simulink model "EiH_VFC_Renew_R2021b"  (R2021b)
settings: Solver=ode4  StartTime=0.0  StopTime=30  FixedStep=0.01  RelTol=1e-3
values from neighbouring files (symbols this model uses):
  denomi_threshold = 1e-8    (= 1e-08)    [param_EiH_VFC.m]
  Keo1 = Keo_Gain    (= 0.5)    [param_EiH_VFC.m]
  Keo2 = Keo_Gain    (= 0.5)    [param_EiH_VFC.m]
  Keo3 = Keo_Gain    (= 0.5)    [param_EiH_VFC.m]
  Keo4 = Keo_Gain    (= 0.5)    [param_EiH_VFC.m]
  Keo5 = Keo_Gain    (= 0.5)    [param_EiH_VFC.m]
  Keo6 = Keo_Gain    (= 0.5)    [param_EiH_VFC.m]
  pco_bar_init = pco_init + [0.15; 0.3; -0.1]    [param_EiH_VFC.m]
  pco_init = [0.0; 0.0; -1.0]    [param_EiH_VFC.m]
  Pinho_Para = [0; 0; 0; lambda_mx; lambda_my]    [param_EiH_VFC.m]
  po = [xo1; yo1; zo1; xo2; yo2; zo2; xo3; yo3; zo3; xo4; yo4; zo4]    [param_EiH_VFC.m]
  pzeta_wo_init = [pwo_init;zetawo_init]    [param_EiH_VFC.m]
  R_threshold = 1e-8    (= 1e-08)    [param_EiH_VFC.m]
  Rco_bar_init = Rfromxi(zetaco_bar_init)    [param_EiH_VFC.m]
  Rco_init = Rfromxi(zetaco_init)    [param_EiH_VFC.m]
  sx = -1.02500e5    (= -102500)    [param_EiH_VFC.m]
  sy = -1.02500e5    (= -102500)    [param_EiH_VFC.m]
  zeta_threshold = 1e-8    (= 1e-08)    [param_EiH_VFC.m]
undefined symbols (not defined in the file or in its folder): Angle, Axis, Km1, Km2, Km3, Km4, Km5, Km6, magnitude, pzeta_md
libraries: dspmtrx3 x2, robotcorelib x1, vrlib x1
(part 4 of 4)

== system EiH_VFC_Renew_R2021b/Image Jacobian fco/Image Jacobian/J3/Ji_Left/Ji_Left_x ==
  pci_bar : Inport
  Pinho_Para : Inport  Port=2
  Demux2 : Demux  Outputs=3
      settings: DisplayOption=none
  Demux4 : Demux  Outputs=5
      settings: DisplayOption=none
  Product1 : Product  Inputs=4  InputSameDT=on  SaturateOnIntegerOverflow=on  OutDataTypeStr=Inherit: Same as first input
  Product2 : Product  Inputs=/  InputSameDT=on  SaturateOnIntegerOverflow=on  OutDataTypeStr=Inherit: Same as first input
  Product3 : Product  Inputs=4  InputSameDT=on  SaturateOnIntegerOverflow=on  OutDataTypeStr=Inherit: Same as first input
  Sum : Sum  InputSameDT=on  SaturateOnIntegerOverflow=on  OutDataTypeStr=Inherit: Same as first input
  Terminator{,1..4} (5 alike) : Terminator
  constant1 : Constant  Value=[0;1]  VectorParams1D=off
  constant2 : Constant  Value=[1;0]  VectorParams1D=off
  constant3 : Constant  VectorParams1D=off
  constant4 : Constant  Value=0  VectorParams1D=off
  denomi_threshold : Subsystem
  Ji_Left_x : Outport  VectorParamsAs1DForOutWhenUnconnected=off
  wires:
  Demux2/3 -> denomi_threshold/1(0)
  Demux4/5 -> Product1/1
  Demux4/3 -> Terminator4/1
  Demux2/1 -> Terminator3/1
  constant4/1 -> Product1/4
  constant3/1 -> Product3/4
  Product2/1 -> Product1/3, Product3/3
  constant1/1 -> Product1/2
  Sum/1 -> Ji_Left_x/1
  Demux4/4 -> Product3/1
  Demux4/2 -> Terminator1/1
  Demux4/1 -> Terminator/1
  denomi_threshold/1(not 0) -> Product2/1
  constant2/1 -> Product3/2
  Product3/1 -> Sum/1
  Product1/1 -> Sum/2
  pci_bar/1 -> Demux2/1
  Pinho_Para/1 -> Demux4/1
  Demux2/2 -> Terminator2/1

== system EiH_VFC_Renew_R2021b/Image Jacobian fco/Image Jacobian/J3/Ji_Left/Ji_Left_y ==
  pci_bar : Inport
  Pinho_Para : Inport  Port=2
  Demux2 : Demux  Outputs=3
      settings: DisplayOption=none
  Demux4 : Demux  Outputs=5
      settings: DisplayOption=none
  Product1 : Product  Inputs=4  InputSameDT=on  SaturateOnIntegerOverflow=on  OutDataTypeStr=Inherit: Same as first input
  Product2 : Product  Inputs=/  InputSameDT=on  SaturateOnIntegerOverflow=on  OutDataTypeStr=Inherit: Same as first input
  Product3 : Product  Inputs=4  InputSameDT=on  SaturateOnIntegerOverflow=on  OutDataTypeStr=Inherit: Same as first input
  Sum : Sum  InputSameDT=on  SaturateOnIntegerOverflow=on  OutDataTypeStr=Inherit: Same as first input
  Terminator{,1..4} (5 alike) : Terminator
  constant1 : Constant  Value=[0;1]  VectorParams1D=off
  constant2 : Constant  Value=[1;0]  VectorParams1D=off
  constant3 : Constant  Value=0  VectorParams1D=off
  constant4 : Constant  VectorParams1D=off
  denomi_threshold : Subsystem
  Ji_Left_y : Outport  VectorParamsAs1DForOutWhenUnconnected=off
  wires:
  Product1/1 -> Sum/2
  Product3/1 -> Sum/1
  constant2/1 -> Product3/2
  denomi_threshold/1(not 0) -> Product2/1
  Demux4/1 -> Terminator/1
  Demux4/2 -> Terminator1/1
  Demux4/4 -> Product3/1
  pci_bar/1 -> Demux2/1
  Sum/1 -> Ji_Left_y/1
  Pinho_Para/1 -> Demux4/1
  constant1/1 -> Product1/2
  Product2/1 -> Product3/3, Product1/3
  constant3/1 -> Product3/4
  constant4/1 -> Product1/4
  Demux2/1 -> Terminator3/1
  Demux4/3 -> Terminator4/1
  Demux4/5 -> Product1/1
  Demux2/3 -> denomi_threshold/1(0)
  Demux2/2 -> Terminator2/1

== system EiH_VFC_Renew_R2021b/Image Jacobian fco/Image Jacobian/J3/Ji_Left/Ji_Left_z ==
  pci_bar : Inport
  Pinho_Para : Inport  Port=2
  Demux2 : Demux  Outputs=3
      settings: DisplayOption=none
  Demux4 : Demux  Outputs=5
      settings: DisplayOption=none
  Product1 : Product  Inputs=5  InputSameDT=on  SaturateOnIntegerOverflow=on  OutDataTypeStr=Inherit: Same as first input
  Product2 : Product  Inputs=/  InputSameDT=on  SaturateOnIntegerOverflow=on  OutDataTypeStr=Inherit: Same as first input
  Product3 : Product  Inputs=5  InputSameDT=on  SaturateOnIntegerOverflow=on  OutDataTypeStr=Inherit: Same as first input
  Sum : Sum  Inputs=--  InputSameDT=on  SaturateOnIntegerOverflow=on  OutDataTypeStr=Inherit: Same as first input
  Terminator : Terminator
  Terminator1 : Terminator
  Terminator2 : Terminator
  constant1 : Constant  Value=[0;1]  VectorParams1D=off
  constant2 : Constant  Value=[1;0]  VectorParams1D=off
  denomi_threshold : Subsystem
  Ji_Left_z : Outport  VectorParamsAs1DForOutWhenUnconnected=off
  wires:
  Demux2/1 -> Product3/2
  Product2/1 -> Product3/5, Product3/4, Product1/4, Product1/5
  constant1/1 -> Product1/3
  Pinho_Para/1 -> Demux4/1
  Sum/1 -> Ji_Left_z/1
  pci_bar/1 -> Demux2/1
  Demux4/4 -> Product3/1
  Demux4/2 -> Terminator1/1
  Demux4/1 -> Terminator/1
  denomi_threshold/1(not 0) -> Product2/1
  constant2/1 -> Product3/3
  Product3/1 -> Sum/1
  Product1/1 -> Sum/2
  Demux4/3 -> Terminator2/1
  Demux4/5 -> Product1/1
  Demux2/3 -> denomi_threshold/1(0)
  Demux2/2 -> Product1/2

== system EiH_VFC_Renew_R2021b/Image Jacobian fco/Image Jacobian/J3/Ji_Right/wedge ==
  "[3x1]" : Inport
  Product1 : Product  InputSameDT=on  SaturateOnIntegerOverflow=on  OutDataTypeStr=Inherit: Same as first input
  Product2 : Product  InputSameDT=on  SaturateOnIntegerOverflow=on  OutDataTypeStr=Inherit: Same as first input
  Product3 : Product  InputSameDT=on  SaturateOnIntegerOverflow=on  OutDataTypeStr=Inherit: Same as first input
  Sum : Sum  Inputs=+++  InputSameDT=on  SaturateOnIntegerOverflow=on  OutDataTypeStr=Inherit: Same as first input
  Xaxis : Constant  Value=[0 0 0;0 0 -1;0 1 0]  VectorParams1D=off
  Yaxis : Constant  Value=[0 0 1;0 0 0;-1 0 0]  VectorParams1D=off
  Zaxis : Constant  Value=[0 -1 0;1 0 0;0 0 0]  VectorParams1D=off
  x : Gain  Gain=[1 0 0]  Multiplication=Matrix(K*u)  SaturateOnIntegerOverflow=on  OutDataTypeStr=Inherit: Same as input  ParamDataTypeStr=Inherit: Same as input
  y : Gain  Gain=[0 1 0]  Multiplication=Matrix(K*u)  SaturateOnIntegerOverflow=on  OutDataTypeStr=Inherit: Same as input  ParamDataTypeStr=Inherit: Same as input
  z : Gain  Gain=[0 0 1]  Multiplication=Matrix(K*u)  SaturateOnIntegerOverflow=on  OutDataTypeStr=Inherit: Same as input  ParamDataTypeStr=Inherit: Same as input
  "[3x3]" : Outport  VectorParamsAs1DForOutWhenUnconnected=off
  wires:
  Zaxis/1 -> Product1/2
  z/1 -> Product1/1
  Xaxis/1 -> Product2/2
  x/1 -> Product2/1
  Yaxis/1 -> Product3/2
  y/1 -> Product3/1
  "[3x1]"/1 -> y/1, x/1, z/1
  Product3/1 -> Sum/2
  Product2/1 -> Sum/1
  Product1/1 -> Sum/3
  Sum/1 -> "[3x3]"/1

== system EiH_VFC_Renew_R2021b/Image Jacobian fco/Image Jacobian/J4/Ji_Left/Ji_Left_x ==
  pci_bar : Inport
  Pinho_Para : Inport  Port=2
  Demux2 : Demux  Outputs=3
      settings: DisplayOption=none
  Demux4 : Demux  Outputs=5
      settings: DisplayOption=none
  Product1 : Product  Inputs=4  InputSameDT=on  SaturateOnIntegerOverflow=on  OutDataTypeStr=Inherit: Same as first input
  Product2 : Product  Inputs=/  InputSameDT=on  SaturateOnIntegerOverflow=on  OutDataTypeStr=Inherit: Same as first input
  Product3 : Product  Inputs=4  InputSameDT=on  SaturateOnIntegerOverflow=on  OutDataTypeStr=Inherit: Same as first input
  Sum : Sum  InputSameDT=on  SaturateOnIntegerOverflow=on  OutDataTypeStr=Inherit: Same as first input
  Terminator{,1..4} (5 alike) : Terminator
  constant1 : Constant  Value=[0;1]  VectorParams1D=off
  constant2 : Constant  Value=[1;0]  VectorParams1D=off
  constant3 : Constant  VectorParams1D=off
  constant4 : Constant  Value=0  VectorParams1D=off
  denomi_threshold : Subsystem
  Ji_Left_x : Outport  VectorParamsAs1DForOutWhenUnconnected=off
  wires:
  Demux2/3 -> denomi_threshold/1(0)
  Demux4/5 -> Product1/1
  Demux4/3 -> Terminator4/1
  Demux2/1 -> Terminator3/1
  constant4/1 -> Product1/4
  constant3/1 -> Product3/4
  Product2/1 -> Product1/3, Product3/3
  constant1/1 -> Product1/2
  Sum/1 -> Ji_Left_x/1
  Demux4/4 -> Product3/1
  Demux4/2 -> Terminator1/1
  Demux4/1 -> Terminator/1
  denomi_threshold/1(not 0) -> Product2/1
  constant2/1 -> Product3/2
  Product3/1 -> Sum/1
  Product1/1 -> Sum/2
  pci_bar/1 -> Demux2/1
  Pinho_Para/1 -> Demux4/1
  Demux2/2 -> Terminator2/1

== system EiH_VFC_Renew_R2021b/Image Jacobian fco/Image Jacobian/J4/Ji_Left/Ji_Left_y ==
  pci_bar : Inport
  Pinho_Para : Inport  Port=2
  Demux2 : Demux  Outputs=3
      settings: DisplayOption=none
  Demux4 : Demux  Outputs=5
      settings: DisplayOption=none
  Product1 : Product  Inputs=4  InputSameDT=on  SaturateOnIntegerOverflow=on  OutDataTypeStr=Inherit: Same as first input
  Product2 : Product  Inputs=/  InputSameDT=on  SaturateOnIntegerOverflow=on  OutDataTypeStr=Inherit: Same as first input
  Product3 : Product  Inputs=4  InputSameDT=on  SaturateOnIntegerOverflow=on  OutDataTypeStr=Inherit: Same as first input
  Sum : Sum  InputSameDT=on  SaturateOnIntegerOverflow=on  OutDataTypeStr=Inherit: Same as first input
  Terminator{,1..4} (5 alike) : Terminator
  constant1 : Constant  Value=[0;1]  VectorParams1D=off
  constant2 : Constant  Value=[1;0]  VectorParams1D=off
  constant3 : Constant  Value=0  VectorParams1D=off
  constant4 : Constant  VectorParams1D=off
  denomi_threshold : Subsystem
  Ji_Left_y : Outport  VectorParamsAs1DForOutWhenUnconnected=off
  wires:
  Product1/1 -> Sum/2
  Product3/1 -> Sum/1
  constant2/1 -> Product3/2
  denomi_threshold/1(not 0) -> Product2/1
  Demux4/1 -> Terminator/1
  Demux4/2 -> Terminator1/1
  Demux4/4 -> Product3/1
  pci_bar/1 -> Demux2/1
  Sum/1 -> Ji_Left_y/1
  Pinho_Para/1 -> Demux4/1
  constant1/1 -> Product1/2
  Product2/1 -> Product3/3, Product1/3
  constant3/1 -> Product3/4
  constant4/1 -> Product1/4
  Demux2/1 -> Terminator3/1
  Demux4/3 -> Terminator4/1
  Demux4/5 -> Product1/1
  Demux2/3 -> denomi_threshold/1(0)
  Demux2/2 -> Terminator2/1

== system EiH_VFC_Renew_R2021b/Image Jacobian fco/Image Jacobian/J4/Ji_Left/Ji_Left_z ==
  pci_bar : Inport
  Pinho_Para : Inport  Port=2
  Demux2 : Demux  Outputs=3
      settings: DisplayOption=none
  Demux4 : Demux  Outputs=5
      settings: DisplayOption=none
  Product1 : Product  Inputs=5  InputSameDT=on  SaturateOnIntegerOverflow=on  OutDataTypeStr=Inherit: Same as first input
  Product2 : Product  Inputs=/  InputSameDT=on  SaturateOnIntegerOverflow=on  OutDataTypeStr=Inherit: Same as first input
  Product3 : Product  Inputs=5  InputSameDT=on  SaturateOnIntegerOverflow=on  OutDataTypeStr=Inherit: Same as first input
  Sum : Sum  Inputs=--  InputSameDT=on  SaturateOnIntegerOverflow=on  OutDataTypeStr=Inherit: Same as first input
  Terminator : Terminator
  Terminator1 : Terminator
  Terminator2 : Terminator
  constant1 : Constant  Value=[0;1]  VectorParams1D=off
  constant2 : Constant  Value=[1;0]  VectorParams1D=off
  denomi_threshold : Subsystem
  Ji_Left_z : Outport  VectorParamsAs1DForOutWhenUnconnected=off
  wires:
  Demux2/1 -> Product3/2
  Product2/1 -> Product3/5, Product3/4, Product1/4, Product1/5
  constant1/1 -> Product1/3
  Pinho_Para/1 -> Demux4/1
  Sum/1 -> Ji_Left_z/1
  pci_bar/1 -> Demux2/1
  Demux4/4 -> Product3/1
  Demux4/2 -> Terminator1/1
  Demux4/1 -> Terminator/1
  denomi_threshold/1(not 0) -> Product2/1
  constant2/1 -> Product3/3
  Product3/1 -> Sum/1
  Product1/1 -> Sum/2
  Demux4/3 -> Terminator2/1
  Demux4/5 -> Product1/1
  Demux2/3 -> denomi_threshold/1(0)
  Demux2/2 -> Product1/2

== system EiH_VFC_Renew_R2021b/Image Jacobian fco/Image Jacobian/J4/Ji_Right/wedge ==
  "[3x1]" : Inport
  Product1 : Product  InputSameDT=on  SaturateOnIntegerOverflow=on  OutDataTypeStr=Inherit: Same as first input
  Product2 : Product  InputSameDT=on  SaturateOnIntegerOverflow=on  OutDataTypeStr=Inherit: Same as first input
  Product3 : Product  InputSameDT=on  SaturateOnIntegerOverflow=on  OutDataTypeStr=Inherit: Same as first input
  Sum : Sum  Inputs=+++  InputSameDT=on  SaturateOnIntegerOverflow=on  OutDataTypeStr=Inherit: Same as first input
  Xaxis : Constant  Value=[0 0 0;0 0 -1;0 1 0]  VectorParams1D=off
  Yaxis : Constant  Value=[0 0 1;0 0 0;-1 0 0]  VectorParams1D=off
  Zaxis : Constant  Value=[0 -1 0;1 0 0;0 0 0]  VectorParams1D=off
  x : Gain  Gain=[1 0 0]  Multiplication=Matrix(K*u)  SaturateOnIntegerOverflow=on  OutDataTypeStr=Inherit: Same as input  ParamDataTypeStr=Inherit: Same as input
  y : Gain  Gain=[0 1 0]  Multiplication=Matrix(K*u)  SaturateOnIntegerOverflow=on  OutDataTypeStr=Inherit: Same as input  ParamDataTypeStr=Inherit: Same as input
  z : Gain  Gain=[0 0 1]  Multiplication=Matrix(K*u)  SaturateOnIntegerOverflow=on  OutDataTypeStr=Inherit: Same as input  ParamDataTypeStr=Inherit: Same as input
  "[3x3]" : Outport  VectorParamsAs1DForOutWhenUnconnected=off
  wires:
  Zaxis/1 -> Product1/2
  z/1 -> Product1/1
  Xaxis/1 -> Product2/2
  x/1 -> Product2/1
  Yaxis/1 -> Product3/2
  y/1 -> Product3/1
  "[3x1]"/1 -> y/1, x/1, z/1
  Product3/1 -> Sum/2
  Product2/1 -> Sum/1
  Product1/1 -> Sum/3
  Sum/1 -> "[3x3]"/1

== system EiH_VFC_Renew_R2021b/Vision Camera fco/ fcq /fcq1/make fcqi/denomi_threshold ==
  0 : Inport
  Abs : Abs  SaturateOnIntegerOverflow=on
  Switch : Switch  Threshold=denomi_threshold  SaturateOnIntegerOverflow=on  InputSameDT=on
  denomi_threshold : Constant  Value=denomi_threshold  VectorParams1D=off
  not 0 : Outport  VectorParamsAs1DForOutWhenUnconnected=off
  wires:
  Switch/1 -> not 0/1
  denomi_threshold/1 -> Switch/3
  0/1 -> Switch/1, Abs/1
  Abs/1 -> Switch/2

== system EiH_VFC_Renew_R2021b/Vision Camera fco/ fcq /fcq2/make fcqi/denomi_threshold ==
  0 : Inport
  Abs : Abs  SaturateOnIntegerOverflow=on
  Switch : Switch  Threshold=denomi_threshold  SaturateOnIntegerOverflow=on  InputSameDT=on
  denomi_threshold : Constant  Value=denomi_threshold  VectorParams1D=off
  not 0 : Outport  VectorParamsAs1DForOutWhenUnconnected=off
  wires:
  Switch/1 -> not 0/1
  denomi_threshold/1 -> Switch/3
  0/1 -> Switch/1, Abs/1
  Abs/1 -> Switch/2

== system EiH_VFC_Renew_R2021b/Vision Camera fco/ fcq /fcq3/make fcqi/denomi_threshold ==
  0 : Inport
  Abs : Abs  SaturateOnIntegerOverflow=on
  Switch : Switch  Threshold=denomi_threshold  SaturateOnIntegerOverflow=on  InputSameDT=on
  denomi_threshold : Constant  Value=denomi_threshold  VectorParams1D=off
  not 0 : Outport  VectorParamsAs1DForOutWhenUnconnected=off
  wires:
  Switch/1 -> not 0/1
  denomi_threshold/1 -> Switch/3
  0/1 -> Switch/1, Abs/1
  Abs/1 -> Switch/2

== system EiH_VFC_Renew_R2021b/Vision Camera fco/ fcq /fcq4/make fcqi/denomi_threshold ==
  0 : Inport
  Abs : Abs  SaturateOnIntegerOverflow=on
  Switch : Switch  Threshold=denomi_threshold  SaturateOnIntegerOverflow=on  InputSameDT=on
  denomi_threshold : Constant  Value=denomi_threshold  VectorParams1D=off
  not 0 : Outport  VectorParamsAs1DForOutWhenUnconnected=off
  wires:
  Switch/1 -> not 0/1
  denomi_threshold/1 -> Switch/3
  0/1 -> Switch/1, Abs/1
  Abs/1 -> Switch/2

== system EiH_VFC_Renew_R2021b/Vision Camera fco/make pzeta co/Rco -> zeta_co/e_R(R)/sk(R) ==
  R : Inport
  Gain : Gain  Gain=1/2  SaturateOnIntegerOverflow=on  OutDataTypeStr=Inherit: Same as input  ParamDataTypeStr=Inherit: Same as input
  Math Function2 : Math  Operator=transpose  SignedPower=on  SaturateOnIntegerOverflow=on
  Sum : Sum  Inputs=|+-  InputSameDT=on  SaturateOnIntegerOverflow=on  OutDataTypeStr=Inherit: Same as first input
  sk(R) : Outport  VectorParamsAs1DForOutWhenUnconnected=off
  wires:
  R/1 -> Math Function2/1, Sum/1
  Math Function2/1 -> Sum/2
  Sum/1 -> Gain/1
  Gain/1 -> sk(R)/1

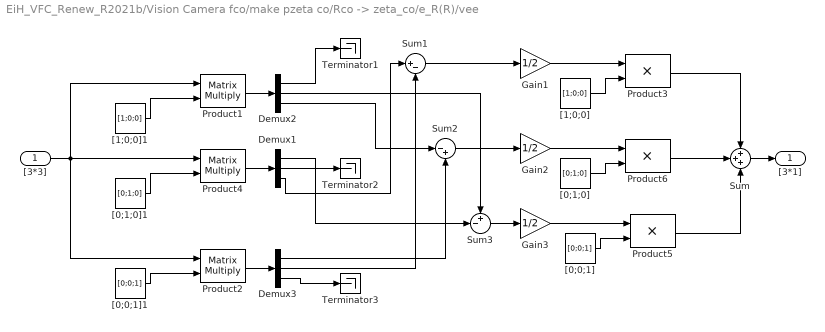
== system EiH_VFC_Renew_R2021b/Vision Camera fco/make pzeta co/Rco -> zeta_co/e_R(R)/vee ==
  "[3*3]" : Inport
  Demux1 : Demux  Outputs=3
      settings: DisplayOption=none
  Demux2 : Demux  Outputs=3
      settings: DisplayOption=none
  Demux3 : Demux  Outputs=3
      settings: DisplayOption=none
  Gain1 : Gain  Gain=1/2  SaturateOnIntegerOverflow=on  OutDataTypeStr=Inherit: Same as input  ParamDataTypeStr=Inherit: Same as input
  Gain2 : Gain  Gain=1/2  SaturateOnIntegerOverflow=on  OutDataTypeStr=Inherit: Same as input  ParamDataTypeStr=Inherit: Same as input
  Gain3 : Gain  Gain=1/2  SaturateOnIntegerOverflow=on  OutDataTypeStr=Inherit: Same as input  ParamDataTypeStr=Inherit: Same as input
  Product1 : Product  Multiplication=Matrix(*)  InputSameDT=on  SaturateOnIntegerOverflow=on  OutDataTypeStr=Inherit: Same as first input
  Product2 : Product  Multiplication=Matrix(*)  InputSameDT=on  SaturateOnIntegerOverflow=on  OutDataTypeStr=Inherit: Same as first input
  Product3 : Product  InputSameDT=on  SaturateOnIntegerOverflow=on  OutDataTypeStr=Inherit: Same as first input
  Product4 : Product  Multiplication=Matrix(*)  InputSameDT=on  SaturateOnIntegerOverflow=on  OutDataTypeStr=Inherit: Same as first input
  Product5 : Product  InputSameDT=on  SaturateOnIntegerOverflow=on  OutDataTypeStr=Inherit: Same as first input
  Product6 : Product  InputSameDT=on  SaturateOnIntegerOverflow=on  OutDataTypeStr=Inherit: Same as first input
  Sum : Sum  Inputs=+++  InputSameDT=on  SaturateOnIntegerOverflow=on  OutDataTypeStr=Inherit: Same as first input
  Sum1 : Sum  Inputs=|+-  InputSameDT=on  SaturateOnIntegerOverflow=on  OutDataTypeStr=Inherit: Same as first input
  Sum2 : Sum  Inputs=|-+  InputSameDT=on  SaturateOnIntegerOverflow=on  OutDataTypeStr=Inherit: Same as first input
  Sum3 : Sum  Inputs=+-|  InputSameDT=on  SaturateOnIntegerOverflow=on  OutDataTypeStr=Inherit: Same as first input
  Terminator1 : Terminator
  Terminator2 : Terminator
  Terminator3 : Terminator
  "[0;0;1]" : Constant  Value=[0;0;1]  VectorParams1D=off
  "[0;0;1]1" : Constant  Value=[0;0;1]  VectorParams1D=off
  "[0;1;0]" : Constant  Value=[0;1;0]  VectorParams1D=off
  "[0;1;0]1" : Constant  Value=[0;1;0]  VectorParams1D=off
  "[1;0;0]" : Constant  Value=[1;0;0]  VectorParams1D=off
  "[1;0;0]1" : Constant  Value=[1;0;0]  VectorParams1D=off
  "[3*1]" : Outport  VectorParamsAs1DForOutWhenUnconnected=off
  wires:
  "[3*3]"/1 -> Product2/1, Product1/1, Product4/1
  "[0;1;0]1"/1 -> Product4/2
  Product4/1 -> Demux1/1
  Demux1/2 -> Terminator2/1
  Demux1/3 -> Sum1/1
  "[1;0;0]1"/1 -> Product1/2
  Product1/1 -> Demux2/1
  Demux2/1 -> Terminator1/1
  "[0;0;1]1"/1 -> Product2/2
  Product2/1 -> Demux3/1
  Demux3/3 -> Terminator3/1
  Demux3/1 -> Sum2/2
  "[1;0;0]"/1 -> Product3/2
  "[0;1;0]"/1 -> Product6/2
  "[0;0;1]"/1 -> Product5/2
  Product6/1 -> Sum/2
  Product5/1 -> Sum/3
  Product3/1 -> Sum/1
  Sum/1 -> "[3*1]"/1
  Sum1/1 -> Gain1/1
  Gain1/1 -> Product3/1
  Demux3/2 -> Sum1/2
  Gain2/1 -> Product6/1
  Gain3/1 -> Product5/1
  Demux2/3 -> Sum2/1
  Sum2/1 -> Gain2/1
  Sum3/1 -> Gain3/1
  Demux2/2 -> Sum3/1
  Demux1/1 -> Sum3/2

== system EiH_VFC_Renew_R2021b/Vision Camera fco/make pzeta co/Rco -> zeta_co/make zeta/3x1 -> 2norm ==
  3x1 : Inport
  Demux : Demux  Outputs=3
      settings: DisplayOption=none
  Math Function : Math  Operator=magnitude^2  SignedPower=on  SaturateOnIntegerOverflow=on
  Math Function1 : Math  Operator=sqrt  SignedPower=on  SaturateOnIntegerOverflow=on
  Sum : Sum  Inputs=+++  InputSameDT=on  SaturateOnIntegerOverflow=on  OutDataTypeStr=Inherit: Same as first input
  2 norm : Outport  VectorParamsAs1DForOutWhenUnconnected=off
  wires:
  Math Function/1 -> Demux/1
  Demux/3 -> Sum/3
  Demux/2 -> Sum/2
  Demux/1 -> Sum/1
  Sum/1 -> Math Function1/1
  Math Function1/1 -> 2 norm/1
  3x1/1 -> Math Function/1

== system EiH_VFC_Renew_R2021b/Vision Camera fco/make pzeta co/Rco -> zeta_co/make zeta/zero check zeta_threshold ==
  In1 : Inport
  Switch : Switch  Threshold=zeta_threshold  SaturateOnIntegerOverflow=on  InputSameDT=on
  norm_eR : Constant  Value=zeta_threshold  VectorParams1D=off
  Out1 : Outport  VectorParamsAs1DForOutWhenUnconnected=off
  wires:
  norm_eR/1 -> Switch/3
  In1/1 -> Switch/1, Switch/2
  Switch/1 -> Out1/1

== system EiH_VFC_Renew_R2021b/make Rco pco/make p_zeta co/make zeta_co/e_R(R)/sk(R) ==
  R : Inport
  Gain : Gain  Gain=1/2  SaturateOnIntegerOverflow=on  OutDataTypeStr=Inherit: Same as input  ParamDataTypeStr=Inherit: Same as input
  Math Function2 : Math  Operator=transpose  SignedPower=on  SaturateOnIntegerOverflow=on
  Sum : Sum  Inputs=|+-  InputSameDT=on  SaturateOnIntegerOverflow=on  OutDataTypeStr=Inherit: Same as first input
  sk(R) : Outport  VectorParamsAs1DForOutWhenUnconnected=off
  wires:
  R/1 -> Math Function2/1, Sum/1
  Math Function2/1 -> Sum/2
  Sum/1 -> Gain/1
  Gain/1 -> sk(R)/1

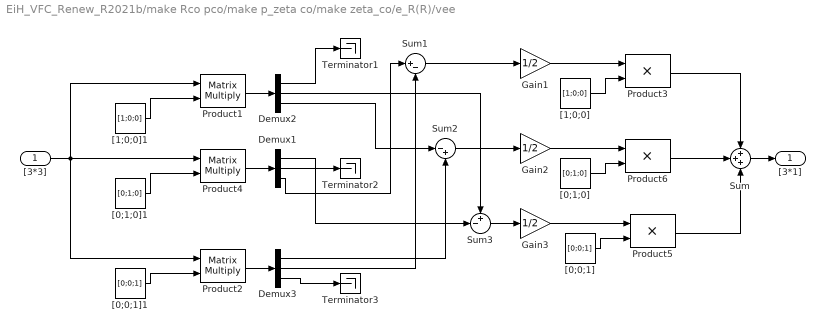
== system EiH_VFC_Renew_R2021b/make Rco pco/make p_zeta co/make zeta_co/e_R(R)/vee ==
  "[3*3]" : Inport
  Demux1 : Demux  Outputs=3
      settings: DisplayOption=none
  Demux2 : Demux  Outputs=3
      settings: DisplayOption=none
  Demux3 : Demux  Outputs=3
      settings: DisplayOption=none
  Gain1 : Gain  Gain=1/2  SaturateOnIntegerOverflow=on  OutDataTypeStr=Inherit: Same as input  ParamDataTypeStr=Inherit: Same as input
  Gain2 : Gain  Gain=1/2  SaturateOnIntegerOverflow=on  OutDataTypeStr=Inherit: Same as input  ParamDataTypeStr=Inherit: Same as input
  Gain3 : Gain  Gain=1/2  SaturateOnIntegerOverflow=on  OutDataTypeStr=Inherit: Same as input  ParamDataTypeStr=Inherit: Same as input
  Product1 : Product  Multiplication=Matrix(*)  InputSameDT=on  SaturateOnIntegerOverflow=on  OutDataTypeStr=Inherit: Same as first input
  Product2 : Product  Multiplication=Matrix(*)  InputSameDT=on  SaturateOnIntegerOverflow=on  OutDataTypeStr=Inherit: Same as first input
  Product3 : Product  InputSameDT=on  SaturateOnIntegerOverflow=on  OutDataTypeStr=Inherit: Same as first input
  Product4 : Product  Multiplication=Matrix(*)  InputSameDT=on  SaturateOnIntegerOverflow=on  OutDataTypeStr=Inherit: Same as first input
  Product5 : Product  InputSameDT=on  SaturateOnIntegerOverflow=on  OutDataTypeStr=Inherit: Same as first input
  Product6 : Product  InputSameDT=on  SaturateOnIntegerOverflow=on  OutDataTypeStr=Inherit: Same as first input
  Sum : Sum  Inputs=+++  InputSameDT=on  SaturateOnIntegerOverflow=on  OutDataTypeStr=Inherit: Same as first input
  Sum1 : Sum  Inputs=|+-  InputSameDT=on  SaturateOnIntegerOverflow=on  OutDataTypeStr=Inherit: Same as first input
  Sum2 : Sum  Inputs=|-+  InputSameDT=on  SaturateOnIntegerOverflow=on  OutDataTypeStr=Inherit: Same as first input
  Sum3 : Sum  Inputs=+-|  InputSameDT=on  SaturateOnIntegerOverflow=on  OutDataTypeStr=Inherit: Same as first input
  Terminator1 : Terminator
  Terminator2 : Terminator
  Terminator3 : Terminator
  "[0;0;1]" : Constant  Value=[0;0;1]  VectorParams1D=off
  "[0;0;1]1" : Constant  Value=[0;0;1]  VectorParams1D=off
  "[0;1;0]" : Constant  Value=[0;1;0]  VectorParams1D=off
  "[0;1;0]1" : Constant  Value=[0;1;0]  VectorParams1D=off
  "[1;0;0]" : Constant  Value=[1;0;0]  VectorParams1D=off
  "[1;0;0]1" : Constant  Value=[1;0;0]  VectorParams1D=off
  "[3*1]" : Outport  VectorParamsAs1DForOutWhenUnconnected=off
  wires:
  "[3*3]"/1 -> Product2/1, Product1/1, Product4/1
  "[0;1;0]1"/1 -> Product4/2
  Product4/1 -> Demux1/1
  Demux1/2 -> Terminator2/1
  Demux1/3 -> Sum1/1
  "[1;0;0]1"/1 -> Product1/2
  Product1/1 -> Demux2/1
  Demux2/1 -> Terminator1/1
  "[0;0;1]1"/1 -> Product2/2
  Product2/1 -> Demux3/1
  Demux3/3 -> Terminator3/1
  Demux3/1 -> Sum2/2
  "[1;0;0]"/1 -> Product3/2
  "[0;1;0]"/1 -> Product6/2
  "[0;0;1]"/1 -> Product5/2
  Product6/1 -> Sum/2
  Product5/1 -> Sum/3
  Product3/1 -> Sum/1
  Sum/1 -> "[3*1]"/1
  Sum1/1 -> Gain1/1
  Gain1/1 -> Product3/1
  Demux3/2 -> Sum1/2
  Gain2/1 -> Product6/1
  Gain3/1 -> Product5/1
  Demux2/3 -> Sum2/1
  Sum2/1 -> Gain2/1
  Sum3/1 -> Gain3/1
  Demux2/2 -> Sum3/1
  Demux1/1 -> Sum3/2

== system EiH_VFC_Renew_R2021b/make Rco pco/make p_zeta co/make zeta_co/make zeta/3x1 -> 2norm ==
  3x1 : Inport
  Demux : Demux  Outputs=3
      settings: DisplayOption=none
  Math Function : Math  Operator=magnitude^2  SignedPower=on  SaturateOnIntegerOverflow=on
  Math Function1 : Math  Operator=sqrt  SignedPower=on  SaturateOnIntegerOverflow=on
  Sum : Sum  Inputs=+++  InputSameDT=on  SaturateOnIntegerOverflow=on  OutDataTypeStr=Inherit: Same as first input
  2 norm : Outport  VectorParamsAs1DForOutWhenUnconnected=off
  wires:
  Math Function/1 -> Demux/1
  Demux/3 -> Sum/3
  Demux/2 -> Sum/2
  Demux/1 -> Sum/1
  Sum/1 -> Math Function1/1
  Math Function1/1 -> 2 norm/1
  3x1/1 -> Math Function/1

== system EiH_VFC_Renew_R2021b/make Rco pco/make p_zeta co/make zeta_co/make zeta/zero check zeta_threshold ==
  In1 : Inport
  Switch : Switch  Threshold=zeta_threshold  SaturateOnIntegerOverflow=on  InputSameDT=on
  norm_eR : Constant  Value=zeta_threshold  VectorParams1D=off
  Out1 : Outport  VectorParamsAs1DForOutWhenUnconnected=off
  wires:
  norm_eR/1 -> Switch/3
  In1/1 -> Switch/1, Switch/2
  Switch/1 -> Out1/1

== system EiH_VFC_Renew_R2021b/Image Jacobian fco/Image Jacobian/J1/Ji_Left/Ji_Left_x/denomi_threshold ==
  0 : Inport
  Abs : Abs  SaturateOnIntegerOverflow=on
  Switch : Switch  Threshold=denomi_threshold  SaturateOnIntegerOverflow=on  InputSameDT=on
  denomi_threshold : Constant  Value=denomi_threshold  VectorParams1D=off
  not 0 : Outport  VectorParamsAs1DForOutWhenUnconnected=off
  wires:
  Switch/1 -> not 0/1
  denomi_threshold/1 -> Switch/3
  0/1 -> Switch/1, Abs/1
  Abs/1 -> Switch/2

== system EiH_VFC_Renew_R2021b/Image Jacobian fco/Image Jacobian/J1/Ji_Left/Ji_Left_y/denomi_threshold ==
  0 : Inport
  Abs : Abs  SaturateOnIntegerOverflow=on
  Switch : Switch  Threshold=denomi_threshold  SaturateOnIntegerOverflow=on  InputSameDT=on
  denomi_threshold : Constant  Value=denomi_threshold  VectorParams1D=off
  not 0 : Outport  VectorParamsAs1DForOutWhenUnconnected=off
  wires:
  Abs/1 -> Switch/2
  0/1 -> Abs/1, Switch/1
  denomi_threshold/1 -> Switch/3
  Switch/1 -> not 0/1

== system EiH_VFC_Renew_R2021b/Image Jacobian fco/Image Jacobian/J1/Ji_Left/Ji_Left_z/denomi_threshold ==
  0 : Inport
  Abs : Abs  SaturateOnIntegerOverflow=on
  Switch : Switch  Threshold=denomi_threshold  SaturateOnIntegerOverflow=on  InputSameDT=on
  denomi_threshold : Constant  Value=denomi_threshold  VectorParams1D=off
  not 0 : Outport  VectorParamsAs1DForOutWhenUnconnected=off
  wires:
  Switch/1 -> not 0/1
  denomi_threshold/1 -> Switch/3
  0/1 -> Switch/1, Abs/1
  Abs/1 -> Switch/2

== system EiH_VFC_Renew_R2021b/Image Jacobian fco/Image Jacobian/J2/Ji_Left/Ji_Left_x/denomi_threshold ==
  0 : Inport
  Abs : Abs  SaturateOnIntegerOverflow=on
  Switch : Switch  Threshold=denomi_threshold  SaturateOnIntegerOverflow=on  InputSameDT=on
  denomi_threshold : Constant  Value=denomi_threshold  VectorParams1D=off
  not 0 : Outport  VectorParamsAs1DForOutWhenUnconnected=off
  wires:
  Switch/1 -> not 0/1
  denomi_threshold/1 -> Switch/3
  0/1 -> Switch/1, Abs/1
  Abs/1 -> Switch/2

== system EiH_VFC_Renew_R2021b/Image Jacobian fco/Image Jacobian/J2/Ji_Left/Ji_Left_y/denomi_threshold ==
  0 : Inport
  Abs : Abs  SaturateOnIntegerOverflow=on
  Switch : Switch  Threshold=denomi_threshold  SaturateOnIntegerOverflow=on  InputSameDT=on
  denomi_threshold : Constant  Value=denomi_threshold  VectorParams1D=off
  not 0 : Outport  VectorParamsAs1DForOutWhenUnconnected=off
  wires:
  Abs/1 -> Switch/2
  0/1 -> Abs/1, Switch/1
  denomi_threshold/1 -> Switch/3
  Switch/1 -> not 0/1

== system EiH_VFC_Renew_R2021b/Image Jacobian fco/Image Jacobian/J2/Ji_Left/Ji_Left_z/denomi_threshold ==
  0 : Inport
  Abs : Abs  SaturateOnIntegerOverflow=on
  Switch : Switch  Threshold=denomi_threshold  SaturateOnIntegerOverflow=on  InputSameDT=on
  denomi_threshold : Constant  Value=denomi_threshold  VectorParams1D=off
  not 0 : Outport  VectorParamsAs1DForOutWhenUnconnected=off
  wires:
  Switch/1 -> not 0/1
  denomi_threshold/1 -> Switch/3
  0/1 -> Switch/1, Abs/1
  Abs/1 -> Switch/2

== system EiH_VFC_Renew_R2021b/Image Jacobian fco/Image Jacobian/J3/Ji_Left/Ji_Left_x/denomi_threshold ==
  0 : Inport
  Abs : Abs  SaturateOnIntegerOverflow=on
  Switch : Switch  Threshold=denomi_threshold  SaturateOnIntegerOverflow=on  InputSameDT=on
  denomi_threshold : Constant  Value=denomi_threshold  VectorParams1D=off
  not 0 : Outport  VectorParamsAs1DForOutWhenUnconnected=off
  wires:
  Switch/1 -> not 0/1
  denomi_threshold/1 -> Switch/3
  0/1 -> Switch/1, Abs/1
  Abs/1 -> Switch/2

== system EiH_VFC_Renew_R2021b/Image Jacobian fco/Image Jacobian/J3/Ji_Left/Ji_Left_y/denomi_threshold ==
  0 : Inport
  Abs : Abs  SaturateOnIntegerOverflow=on
  Switch : Switch  Threshold=denomi_threshold  SaturateOnIntegerOverflow=on  InputSameDT=on
  denomi_threshold : Constant  Value=denomi_threshold  VectorParams1D=off
  not 0 : Outport  VectorParamsAs1DForOutWhenUnconnected=off
  wires:
  Abs/1 -> Switch/2
  0/1 -> Abs/1, Switch/1
  denomi_threshold/1 -> Switch/3
  Switch/1 -> not 0/1

== system EiH_VFC_Renew_R2021b/Image Jacobian fco/Image Jacobian/J3/Ji_Left/Ji_Left_z/denomi_threshold ==
  0 : Inport
  Abs : Abs  SaturateOnIntegerOverflow=on
  Switch : Switch  Threshold=denomi_threshold  SaturateOnIntegerOverflow=on  InputSameDT=on
  denomi_threshold : Constant  Value=denomi_threshold  VectorParams1D=off
  not 0 : Outport  VectorParamsAs1DForOutWhenUnconnected=off
  wires:
  Switch/1 -> not 0/1
  denomi_threshold/1 -> Switch/3
  0/1 -> Switch/1, Abs/1
  Abs/1 -> Switch/2

== system EiH_VFC_Renew_R2021b/Image Jacobian fco/Image Jacobian/J4/Ji_Left/Ji_Left_x/denomi_threshold ==
  0 : Inport
  Abs : Abs  SaturateOnIntegerOverflow=on
  Switch : Switch  Threshold=denomi_threshold  SaturateOnIntegerOverflow=on  InputSameDT=on
  denomi_threshold : Constant  Value=denomi_threshold  VectorParams1D=off
  not 0 : Outport  VectorParamsAs1DForOutWhenUnconnected=off
  wires:
  Switch/1 -> not 0/1
  denomi_threshold/1 -> Switch/3
  0/1 -> Switch/1, Abs/1
  Abs/1 -> Switch/2

== system EiH_VFC_Renew_R2021b/Image Jacobian fco/Image Jacobian/J4/Ji_Left/Ji_Left_y/denomi_threshold ==
  0 : Inport
  Abs : Abs  SaturateOnIntegerOverflow=on
  Switch : Switch  Threshold=denomi_threshold  SaturateOnIntegerOverflow=on  InputSameDT=on
  denomi_threshold : Constant  Value=denomi_threshold  VectorParams1D=off
  not 0 : Outport  VectorParamsAs1DForOutWhenUnconnected=off
  wires:
  Abs/1 -> Switch/2
  0/1 -> Abs/1, Switch/1
  denomi_threshold/1 -> Switch/3
  Switch/1 -> not 0/1

== system EiH_VFC_Renew_R2021b/Image Jacobian fco/Image Jacobian/J4/Ji_Left/Ji_Left_z/denomi_threshold ==
  0 : Inport
  Abs : Abs  SaturateOnIntegerOverflow=on
  Switch : Switch  Threshold=denomi_threshold  SaturateOnIntegerOverflow=on  InputSameDT=on
  denomi_threshold : Constant  Value=denomi_threshold  VectorParams1D=off
  not 0 : Outport  VectorParamsAs1DForOutWhenUnconnected=off
  wires:
  Switch/1 -> not 0/1
  denomi_threshold/1 -> Switch/3
  0/1 -> Switch/1, Abs/1
  Abs/1 -> Switch/2

== matlab function EiH_VFC_Renew_R2021b/make Vwm/MATLAB Function ==
  data: Ad_ge input; inv_Ad_ge output
function inv_Ad_ge = fcn(Ad_ge)

inv_Ad_ge = inv(Ad_ge);
